simulink model "E55_1030"  (R2019b)
settings: Solver=FixedStepDiscrete  StartTime=0.0  StopTime=10  FixedStep=0.0005  RelTol=1e-3  EnableMultiTasking=on
InitFcn:
  | ecucoder_canfd
  | load('DATA_Plimit.mat')
  | a=0.775;
  | b=0.775;
  | kf=-50000;
  | kr=-50000;
  | m=226+75;
  | Iz=100;
  | u=0.85;
  | g=9.8;
  | L=a+b;
  | xi=0.1;
  | r=0.226;
  | Lw=1.171;
  | Tm=21;
  | i=15.9;
  | Jw=0.504;
  | Pmax=20000;
  | mw=19.3;
  | mb=148.9+75;
  | hg=0.280;
model workspace (MAT data in the model file):
  Initial_Steer_Position = 0
values from neighbouring files (symbols this model uses):
  SOC = [2.5 5 7.5 10 20 30 40 50 60 70 80 90 ... (14 elements, 14x1)]    [DATA_Plimit.mat]
  SOC_Discharge = [2.04592350211 2.57821618825 3.10671863859 3.63118835861 4.15200192786 4.66837694959 5.18149950051 5.69046162564 6.19532286188 6.696400261 7.19347596839 7.68712157998 ... (473 elements, 1x473)]    [DATA_Plimit.mat]
  VOLTAGE = [459.1488 476.0844 485.9448 487.344 492.822 498.8016 503.382 509.1108 518.8128 531.2472 544.5132 558.4656 ... (14 elements, 14x1)]    [DATA_Plimit.mat]
undefined symbols (not defined in the file or in its folder): DiscIntNeverNeededParam, H, HALL10, HALL6, HALL7, HALL8, HALL9, HPWM1, HPWM3, I_AN05_5V, I_AN07_5V, I_AN08_5V, I_AN09_5V, I_AN10_5V, I_SW11_H, I_SW12_H, I_SW13_H, I_SW14_H, I_SW15_H, I_SW16_H, I_SW17_H, I_SW18_H, I_SW19_H, LS1A2, O_HS1A2, O_HS1A8
libraries: ec311lib x152, simulink x92, canmsglib x30, canfdmsglib x2
(part 4 of 6)

== system E55_1030/Function-Call Subsystem2/Subsystem11 ==
  CAN_OK : Inport
  CAN ID : Inport  Port=2
  CAN Msg : Inport  Port=3
  function : TriggerPort  TriggerType=function-call  VariantControl=(inherit)
  Enabled Subsystem : Subsystem  TreatAsAtomicUnit=on
  steer_angle_data : Outport
  wires:
  CAN_OK/1 -> Enabled Subsystem/Enable  "CAN_OK"
  CAN ID/1 -> Enabled Subsystem/1(In1)
  CAN Msg/1 -> Enabled Subsystem/2(In2)
  Enabled Subsystem/1(Angle) -> steer_angle_data/1

== system E55_1030/Function-Call Subsystem2/Subsystem12 ==
  CAN_OK : Inport
  CAN ID : Inport  Port=2
  CAN Msg : Inport  Port=3
  function : TriggerPort  TriggerType=function-call  VariantControl=(inherit)
  Bus Creator : BusCreator  Inputs=4
  Enabled Subsystem : Subsystem  TreatAsAtomicUnit=on
  285_data : Outport
  wires:
  CAN_OK/1 -> Enabled Subsystem/Enable  "CAN_OK"
  CAN ID/1 -> Enabled Subsystem/1(In1)
  CAN Msg/1 -> Enabled Subsystem/2(In2)
  Bus Creator/1 -> 285_data/1
  Enabled Subsystem/1(ErrorInfo) -> Bus Creator/1  "ErrorCode"
  Enabled Subsystem/2(TempIGBT) -> Bus Creator/2  "TempIGBT"
  Enabled Subsystem/3(TempInverter) -> Bus Creator/3  "TempInverter"
  Enabled Subsystem/4(TempMotor) -> Bus Creator/4  "TempMotor"

== system E55_1030/Function-Call Subsystem2/Subsystem15 ==
  acc_x : Inport
  acc_y : Inport  Port=2
  Mux : Mux
  Saturation : Saturate  UpperLimit=1500  LowerLimit=0
  右前载荷 : Subsystem
  右后载荷 : Subsystem
  左前载荷 : Subsystem
  左后载荷 : Subsystem
  Fz : Outport
  wires:
  [acc_x] -> 左前载荷/1(acc_x)
  [acc_y] -> 左前载荷/2(acc_y)
  Mux/1 -> Saturation/1
  [acc_x] -> 右前载荷/1(acc_x)
  [acc_y] -> 右前载荷/2(acc_y)
  [acc_x] -> 左后载荷/1(acc_x)
  [acc_y] -> 左后载荷/2(acc_y)
  [acc_x] -> 右后载荷/1(acc_x)
  [acc_y] -> 右后载荷/2(acc_y)
  左前载荷/1(Fz1) -> Mux/1
  右前载荷/1(Fz2) -> Mux/2
  左后载荷/1(Fz3) -> Mux/3
  右后载荷/1(Fz4) -> Mux/4
  acc_y/1 -> [acc_x]
  acc_x/1 -> [acc_y]
  Saturation/1 -> Fz/1

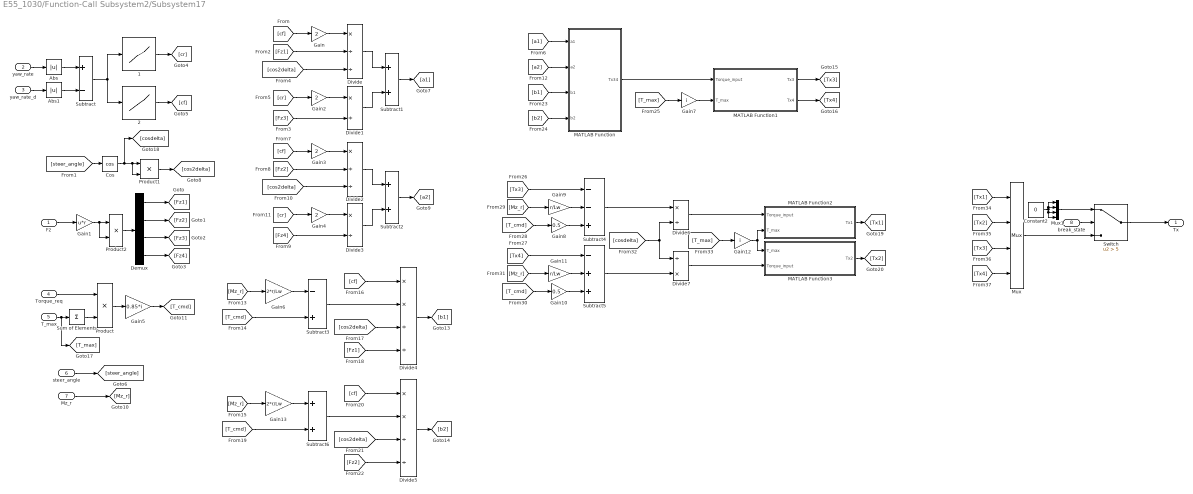
== system E55_1030/Function-Call Subsystem2/Subsystem17 ==
  Fz : Inport
  yaw_rate : Inport  Port=2
  yaw_rate_d : Inport  Port=3
  Torque_req : Inport  Port=4
  T_max : Inport  Port=5
  steer_angle : Inport  Port=6
  Mz_r : Inport  Port=7
  break_state : Inport  Port=8
  1 : Lookup_n-D  NumberOfTableDimensions=1  BreakpointsForDimension1=[-0.3,-0.2,0,0.2,0.3]  Table=[1,1,1,2,2]  InternalRulePriority=Speed  RndMeth=Simplest  InputSameDT=on
  2 : Lookup_n-D  NumberOfTableDimensions=1  BreakpointsForDimension1=[-0.3,-0.2,0,0.2,0.3]  Table=[2,2,1,1,1]  InternalRulePriority=Speed  RndMeth=Simplest  InputSameDT=on
  Abs : Abs
  Abs1 : Abs
  Constant2 : Constant  Value=0
  Cos : Trigonometry  Operator=cos
  Demux : Demux
  Divide : Product  Inputs=*//
  Divide1 : Product  Inputs=*/
  Divide2 : Product  Inputs=*//
  Divide3 : Product  Inputs=*/
  Divide4 : Product  Inputs=**//
  Divide5 : Product  Inputs=**//
  Divide6 : Product  Inputs=*/
  Divide7 : Product  Inputs=/*
  Gain{,2..4} (4 alike) : Gain  Gain=2
  Gain1 : Gain  Gain=u*r
  Gain10 : Gain  Gain=0.5
  Gain11 : Gain  Gain=r/Lw
  Gain12 : Gain  Gain=i
  Gain13 : Gain  Gain=2*r/Lw
  Gain5 : Gain  Gain=0.85*i
  Gain6 : Gain  Gain=2*r/Lw
  Gain7 : Gain  Gain=i
  Gain8 : Gain  Gain=0.5
  Gain9 : Gain  Gain=r/Lw
  MATLAB Function : MATLAB Function  TreatAsAtomicUnit=on
  MATLAB Function1 : MATLAB Function  TreatAsAtomicUnit=on
  MATLAB Function2 : MATLAB Function  TreatAsAtomicUnit=on
  MATLAB Function3 : MATLAB Function  TreatAsAtomicUnit=on
  Mux : Mux
  Mux1 : Mux
  Product : Product
  Product1 : Product
  Product2 : Product
  Subtract : Sum  Inputs=+-
  Subtract1 : Sum
  Subtract2 : Sum
  Subtract3 : Sum  Inputs=-+
  Subtract4 : Sum  Inputs=--+
  Subtract5 : Sum  Inputs=-++
  Subtract6 : Sum
  Sum of Elements : Sum  Inputs=+
  Switch : Switch  Criteria=u2 > Threshold  Threshold=5
  Tx : Outport
  wires:
  Demux/1 -> [Fz1]
  Demux/2 -> [Fz2]
  Demux/3 -> [Fz3]
  Demux/4 -> [Fz4]
  yaw_rate/1 -> Abs/1
  yaw_rate_d/1 -> Abs1/1
  Abs/1 -> Subtract/1
  Abs1/1 -> Subtract/2
  Subtract/1 -> 2/1, 1/1
  [cf] -> Gain/1
  Gain/1 -> Divide/1
  steer_angle/1 -> [steer_angle]
  [steer_angle] -> Cos/1
  [Fz1] -> Divide/2
  Cos/1 -> Product1/2, Product1/1, [cosdelta]
  Product1/1 -> [cos2delta]
  [cos2delta] -> Divide/3
  Divide/1 -> Subtract1/1
  [cr] -> Gain2/1
  Gain2/1 -> Divide1/1
  Fz/1 -> Gain1/1
  [Fz3] -> Divide1/2
  Divide1/1 -> Subtract1/2
  Subtract1/1 -> [a1]
  [a1] -> MATLAB Function/1(a1)
  Subtract2/1 -> [a2]
  Divide3/1 -> Subtract2/2
  [Fz4] -> Divide3/2
  Gain4/1 -> Divide3/1
  [cr] -> Gain4/1
  Divide2/1 -> Subtract2/1
  [cos2delta] -> Divide2/3
  [Fz2] -> Divide2/2
  Gain3/1 -> Divide2/1
  [cf] -> Gain3/1
  [a2] -> MATLAB Function/2(a2)
  Mz_r/1 -> [Mz_r]
  T_max/1 -> [T_max], Sum of Elements/1
  Torque_req/1 -> Product/1
  Product/1 -> Gain5/1
  Gain5/1 -> [T_cmd]
  [Mz_r] -> Gain6/1
  Gain6/1 -> Subtract3/1
  [T_cmd] -> Subtract3/2
  [cf] -> Divide4/1
  [cos2delta] -> Divide4/3
  [Fz1] -> Divide4/4
  Divide4/1 -> [b1]
  Divide5/1 -> [b2]
  [Fz2] -> Divide5/4
  [cos2delta] -> Divide5/3
  [cf] -> Divide5/1
  [b1] -> MATLAB Function/3(b1)
  [b2] -> MATLAB Function/4(b2)
  Sum of Elements/1 -> Product/2
  MATLAB Function/1(Tx34) -> MATLAB Function1/1(Torque_input)
  [T_max] -> Gain7/1
  Gain7/1 -> MATLAB Function1/2(T_max)
  MATLAB Function1/2(Tx4) -> [Tx4]
  MATLAB Function1/1(Tx3) -> [Tx3]
  [T_cmd] -> Gain8/1
  Gain8/1 -> Subtract4/3
  [Mz_r] -> Gain9/1
  [Tx3] -> Subtract4/1
  Gain9/1 -> Subtract4/2
  [Mz_r] -> Gain11/1
  Gain11/1 -> Subtract5/2
  Gain10/1 -> Subtract5/3
  [T_cmd] -> Gain10/1
  [Tx4] -> Subtract5/1
  Subtract4/1 -> Divide6/1
  [cosdelta] -> Divide7/1, Divide6/2
  Subtract5/1 -> Divide7/2
  Divide6/1 -> MATLAB Function2/1(Torque_input)
  [T_max] -> Gain12/1
  Gain12/1 -> MATLAB Function3/1(T_max), MATLAB Function2/2(T_max)
  Divide7/1 -> MATLAB Function3/2(Torque_input)
  MATLAB Function2/1(Tx1) -> [Tx1]
  MATLAB Function3/1(Tx2) -> [Tx2]
  Mux/1 -> Switch/3
  2/1 -> [cf]
  1/1 -> [cr]
  Subtract3/1 -> Divide4/2
  [T_cmd] -> Subtract6/2
  Gain13/1 -> Subtract6/1
  [Mz_r] -> Gain13/1
  Subtract6/1 -> Divide5/2
  break_state/1 -> Switch/2
  Switch/1 -> Tx/1
  Mux1/1 -> Switch/1
  Constant2/1 -> Mux1/3, Mux1/4, Mux1/2, Mux1/1
  [Tx1] -> Mux/1
  [Tx2] -> Mux/2
  [Tx3] -> Mux/3
  [Tx4] -> Mux/4
  Product2/1 -> Demux/1
  Gain1/1 -> Product2/2, Product2/1

== system E55_1030/Function-Call Subsystem2/Subsystem18 ==
  CAN_OK : Inport
  CAN ID : Inport  Port=2
  CAN Msg : Inport  Port=3
  DLC : Inport  Port=4
  function : TriggerPort  TriggerType=function-call  VariantControl=(inherit)
  Bus Creator : BusCreator  Inputs=7
  Enabled Subsystem : Subsystem  TreatAsAtomicUnit=on
  GNSS_data : Outport
  wires:
  CAN_OK/1 -> Enabled Subsystem/Enable, Bus Creator/1  "CAN_OK"
  CAN ID/1 -> Enabled Subsystem/1(In1)
  CAN Msg/1 -> Enabled Subsystem/2(In2)
  Bus Creator/1 -> GNSS_data/1
  DLC/1 -> Enabled Subsystem/3(In3)
  Enabled Subsystem/2(Heading_Angle) -> Bus Creator/3  "Heading_Angle"
  Enabled Subsystem/1(East_Speed) -> Bus Creator/2  "East_Speed"
  Enabled Subsystem/3(North_Speed) -> Bus Creator/4  "North_Speed"
  Enabled Subsystem/4(Pitch_Angle) -> Bus Creator/5  "Pitch_Angle"
  Enabled Subsystem/5(Roll_Angle) -> Bus Creator/6  "Roll_Angle"
  Enabled Subsystem/6(To_Ground_Speed) -> Bus Creator/7  "To_Ground_Speed"

== system E55_1030/Function-Call Subsystem2/Subsystem19 ==
  CAN_OK : Inport
  CAN ID : Inport  Port=2
  CAN Msg : Inport  Port=3
  DLC : Inport  Port=4
  function : TriggerPort  TriggerType=function-call  VariantControl=(inherit)
  Bus Creator : BusCreator  Inputs=7
  Enabled Subsystem : Subsystem  TreatAsAtomicUnit=on
  IMU_data : Outport
  wires:
  CAN_OK/1 -> Enabled Subsystem/Enable, Bus Creator/1  "CAN_OK"
  CAN ID/1 -> Enabled Subsystem/1(In1)
  CAN Msg/1 -> Enabled Subsystem/2(In2)
  Bus Creator/1 -> IMU_data/1
  DLC/1 -> Enabled Subsystem/3(In3)
  Enabled Subsystem/1(INS_IMUAccrnX) -> Bus Creator/2  "INS_IMUAccrnX"
  Enabled Subsystem/2(INS_IMUAccrnY) -> Bus Creator/3  "INS_IMUAccrnY"
  Enabled Subsystem/3(INS_IMUAccrnZ) -> Bus Creator/4  "INS_IMUAccrnZ"
  Enabled Subsystem/4(INS_IMUAglRateX) -> Bus Creator/5  "INS_IMUAglRateX"
  Enabled Subsystem/5(INS_IMUAglRateY) -> Bus Creator/6  "INS_IMUAglRateY"
  Enabled Subsystem/6(INS_IMUAglRateZ) -> Bus Creator/7  "INS_IMUAglRateZ"

== system E55_1030/Function-Call Subsystem2/Subsystem2 ==
  CAN_OK : Inport
  CAN ID : Inport  Port=2
  CAN Msg : Inport  Port=3
  function : TriggerPort  TriggerType=function-call  VariantControl=(inherit)
  Bus Creator : BusCreator  Inputs=4
  Enabled Subsystem : Subsystem  TreatAsAtomicUnit=on
  287_data : Outport
  wires:
  CAN_OK/1 -> Enabled Subsystem/Enable
  CAN ID/1 -> Enabled Subsystem/1(In1)
  CAN Msg/1 -> Enabled Subsystem/2(In2)
  Enabled Subsystem/2(287_Error) -> Bus Creator/2  "bError"
  Enabled Subsystem/1(287_ActualVelocity) -> Bus Creator/1  "AMK_Speed"
  Bus Creator/1 -> 287_data/1
  Enabled Subsystem/3(287_Id) -> Bus Creator/3  "Id"
  Enabled Subsystem/4(287_Iq) -> Bus Creator/4  "Iq"

== system E55_1030/Function-Call Subsystem2/Subsystem3 ==
  CAN_OK : Inport
  CAN ID : Inport  Port=2
  CAN Msg : Inport  Port=3
  function : TriggerPort  TriggerType=function-call  VariantControl=(inherit)
  Bus Creator : BusCreator  Inputs=4
  Enabled Subsystem : Subsystem  TreatAsAtomicUnit=on
  283_data : Outport
  wires:
  CAN_OK/1 -> Enabled Subsystem/Enable
  CAN ID/1 -> Enabled Subsystem/1(In1)
  CAN Msg/1 -> Enabled Subsystem/2(In2)
  Enabled Subsystem/2(283_Error) -> Bus Creator/2  "bError"
  Enabled Subsystem/1(283_ActualVelocity) -> Bus Creator/1  "AMK_Speed"
  Bus Creator/1 -> 283_data/1
  Enabled Subsystem/3(283_Id) -> Bus Creator/3  "Id"
  Enabled Subsystem/4(283_Iq) -> Bus Creator/4  "Iq"

== system E55_1030/Function-Call Subsystem2/Subsystem4 ==
  CAN_OK : Inport
  CAN ID : Inport  Port=2
  CAN Msg : Inport  Port=3
  function : TriggerPort  TriggerType=function-call  VariantControl=(inherit)
  Bus Creator : BusCreator  Inputs=4
  Enabled Subsystem : Subsystem  TreatAsAtomicUnit=on
  288_data : Outport
  wires:
  CAN_OK/1 -> Enabled Subsystem/Enable
  CAN ID/1 -> Enabled Subsystem/1(In1)
  CAN Msg/1 -> Enabled Subsystem/2(In2)
  Enabled Subsystem/2(288_Error) -> Bus Creator/2  "bError"
  Enabled Subsystem/1(288_ActualVelocity) -> Bus Creator/1  "AMK_Speed"
  Bus Creator/1 -> 288_data/1
  Enabled Subsystem/3(288_Id) -> Bus Creator/3  "Id"
  Enabled Subsystem/4(288_Iq) -> Bus Creator/4  "Iq"

== system E55_1030/Function-Call Subsystem2/Subsystem5 ==
  CAN_OK : Inport
  CAN ID : Inport  Port=2
  CAN Msg : Inport  Port=3
  function : TriggerPort  TriggerType=function-call  VariantControl=(inherit)
  Bus Creator : BusCreator  Inputs=4
  Enabled Subsystem : Subsystem  TreatAsAtomicUnit=on
  286_data : Outport
  wires:
  CAN_OK/1 -> Enabled Subsystem/Enable  "CAN_OK"
  CAN ID/1 -> Enabled Subsystem/1(In1)
  CAN Msg/1 -> Enabled Subsystem/2(In2)
  Bus Creator/1 -> 286_data/1
  Enabled Subsystem/1(ErrorInfo) -> Bus Creator/1  "ErrorCode"
  Enabled Subsystem/2(TempIGBT) -> Bus Creator/2  "TempIGBT"
  Enabled Subsystem/3(TempInverter) -> Bus Creator/3  "TempInverter"
  Enabled Subsystem/4(TempMotor) -> Bus Creator/4  "TempMotor"

== system E55_1030/Function-Call Subsystem2/Subsystem6 ==
  CAN_OK : Inport
  CAN ID : Inport  Port=2
  CAN Msg : Inport  Port=3
  function : TriggerPort  TriggerType=function-call  VariantControl=(inherit)
  Bus Creator : BusCreator  Inputs=4
  Enabled Subsystem : Subsystem  TreatAsAtomicUnit=on
  289_data : Outport
  wires:
  CAN_OK/1 -> Enabled Subsystem/Enable  "CAN_OK"
  CAN ID/1 -> Enabled Subsystem/1(In1)
  CAN Msg/1 -> Enabled Subsystem/2(In2)
  Bus Creator/1 -> 289_data/1
  Enabled Subsystem/1(ErrorInfo) -> Bus Creator/1  "ErrorCode"
  Enabled Subsystem/2(TempIGBT) -> Bus Creator/2  "TempIGBT"
  Enabled Subsystem/3(TempInverter) -> Bus Creator/3  "TempInverter"
  Enabled Subsystem/4(TempMotor) -> Bus Creator/4  "TempMotor"

== system E55_1030/Function-Call Subsystem2/Subsystem7 ==
  CAN_OK : Inport
  CAN ID : Inport  Port=2
  CAN Msg : Inport  Port=3
  function : TriggerPort  TriggerType=function-call  VariantControl=(inherit)
  Bus Creator : BusCreator  Inputs=4
  Enabled Subsystem : Subsystem  TreatAsAtomicUnit=on
  28A_data : Outport
  wires:
  CAN_OK/1 -> Enabled Subsystem/Enable  "CAN_OK"
  CAN ID/1 -> Enabled Subsystem/1(In1)
  CAN Msg/1 -> Enabled Subsystem/2(In2)
  Bus Creator/1 -> 28A_data/1
  Enabled Subsystem/1(ErrorInfo) -> Bus Creator/1  "ErrorCode"
  Enabled Subsystem/2(TempIGBT) -> Bus Creator/2  "TempIGBT"
  Enabled Subsystem/3(TempInverter) -> Bus Creator/3  "TempInverter"
  Enabled Subsystem/4(TempMotor) -> Bus Creator/4  "TempMotor"

== system E55_1030/Function-Call Subsystem2/Subsystem8 ==
  CAN_OK : Inport
  CAN ID : Inport  Port=2
  CAN Msg : Inport  Port=3
  function : TriggerPort  TriggerType=function-call  VariantControl=(inherit)
  Bus Creator : BusCreator  Inputs=2
  Enabled Subsystem : Subsystem  TreatAsAtomicUnit=on
  IVT_data : Outport
  wires:
  CAN_OK/1 -> Enabled Subsystem/Enable  "CAN_OK"
  CAN ID/1 -> Enabled Subsystem/1(In1)
  CAN Msg/1 -> Enabled Subsystem/2(In2)
  Bus Creator/1 -> IVT_data/1
  Enabled Subsystem/1(IVT_MsgCount) -> Bus Creator/1  "IVT_MsgCount"
  Enabled Subsystem/2(IVT_Msg_Result_W) -> Bus Creator/2  "IVT_Msg_Result_W"

== system E55_1030/Function-Call Subsystem2/Triggered Subsystem ==
  Trigger : TriggerPort  TriggerType=falling  VariantControl=Variant
  AMK_Setpoints_Motor1 : Subsystem
  AMK_Setpoints_Motor2 : Subsystem
  AMK_Setpoints_Motor3 : Subsystem
  AMK_Setpoints_Motor4 : Subsystem
  Constant{,1..3} (4 alike) : Constant  Value=0
  Constant{4..6,15} (4 alike) : Constant  Value=1792
  Terminator{42..43,48,50} (4 alike) : Terminator
  右前 : ec311lib/RapidECU_U34/03CANCommunication/CAN0to2Transmit  canmodule=2  canbuffer=8  canmessageid=hex2dec('0185')  canmessagetype=Standard(11-bit ID)  datalength=8  sampletime=-1
      settings: SourceProductName=ECUCoder for S32K311
  右后 : ec311lib/RapidECU_U34/03CANCommunication/CAN0to2Transmit  canmodule=2  canbuffer=11  canmessageid=hex2dec('0189')  canmessagetype=Standard(11-bit ID)  datalength=8  sampletime=-1
      settings: SourceProductName=ECUCoder for S32K311
  左前 : ec311lib/RapidECU_U34/03CANCommunication/CAN0to2Transmit  canmodule=2  canbuffer=7  canmessageid=hex2dec('0184')  canmessagetype=Standard(11-bit ID)  datalength=8  sampletime=-1
      settings: SourceProductName=ECUCoder for S32K311
  左后 : ec311lib/RapidECU_U34/03CANCommunication/CAN0to2Transmit  canmodule=2  canbuffer=10  canmessageid=hex2dec('0188')  canmessagetype=Standard(11-bit ID)  datalength=8  sampletime=-1
      settings: SourceProductName=ECUCoder for S32K311
  wires:
  AMK_Setpoints_Motor1/1(output) -> 右前/1
  AMK_Setpoints_Motor3/1(output) -> 左前/1
  右前/1 -> Terminator42/1
  左后/1 -> Terminator48/1
  AMK_Setpoints_Motor2/1(output) -> 左后/1
  左前/1 -> Terminator43/1
  AMK_Setpoints_Motor4/1(output) -> 右后/1
  右后/1 -> Terminator50/1
  Constant/1 -> AMK_Setpoints_Motor1/3(AMK_TargetVelocity_in), AMK_Setpoints_Motor1/1(AMK_TorqueLimitNegativ_in), AMK_Setpoints_Motor1/2(AMK_TorqueLimitPositiv_in)
  Constant1/1 -> AMK_Setpoints_Motor3/3(AMK_TargetVelocity_in), AMK_Setpoints_Motor3/2(AMK_TorqueLimitPositiv_in), AMK_Setpoints_Motor3/1(AMK_TorqueLimitNegativ_in)
  Constant2/1 -> AMK_Setpoints_Motor4/2(AMK_TorqueLimitPositiv_in), AMK_Setpoints_Motor4/3(AMK_TargetVelocity_in), AMK_Setpoints_Motor4/1(AMK_TorqueLimitNegativ_in)
  Constant3/1 -> AMK_Setpoints_Motor2/3(AMK_TargetVelocity_in), AMK_Setpoints_Motor2/2(AMK_TorqueLimitPositiv_in), AMK_Setpoints_Motor2/1(AMK_TorqueLimitNegativ_in)
  Constant15/1 -> AMK_Setpoints_Motor1/4(AMK_Control_in)
  Constant4/1 -> AMK_Setpoints_Motor2/4(AMK_Control_in)
  Constant5/1 -> AMK_Setpoints_Motor3/4(AMK_Control_in)
  Constant6/1 -> AMK_Setpoints_Motor4/4(AMK_Control_in)

== system E55_1030/Function-Call Subsystem2/功率限制 ==
  MaxTempMotor : Inport
  wheel_speed : Inport  Port=2
  "Power " : Inport  Port=3
  1-D Lookup Table1 : Lookup_n-D  NumberOfTableDimensions=1  BreakpointsForDimension1=[0;80;100;120]  Table=[22.3056525;22.3056525;21.8349456;21.3643326]  InternalRulePriority=Speed  RndMeth=Simplest  InputSameDT=on
  Constant : Constant  Value=60/(2*pi)
  Divide1 : Product  Inputs=**/
  Min : MinMax  Inputs=2
  Saturation : Saturate  UpperLimit=20000  LowerLimit=2000
  T_max : Outport
  wires:
  MaxTempMotor/1 -> 1-D Lookup Table1/1
  Divide1/1 -> Min/1
  Min/1 -> T_max/1
  wheel_speed/1 -> Saturation/1
  [T_max_temp] -> Min/2
  1-D Lookup Table1/1 -> [T_max_temp]
  Constant/1 -> Divide1/2
  "Power "/1 -> Divide1/1
  Saturation/1 -> Divide1/3

== system E55_1030/Function-Call Subsystem2/功率限制1 ==
  MaxTempMotor : Inport
  wheel_speed : Inport  Port=2
  DeratingRatio : Inport  Port=3
  1-D Lookup Table1 : Lookup_n-D  NumberOfTableDimensions=1  BreakpointsForDimension1=[0;80;100;120]  Table=[22.3056525;22.3056525;21.8349456;21.3643326]  InternalRulePriority=Speed  RndMeth=Simplest  InputSameDT=on
  Constant : Constant  Value=60*20000/(2*pi)
  Divide1 : Product  Inputs=*/
  Gain : Gain  Gain=i
  Min : MinMax  Inputs=2
  Product : Product
  Saturation : Saturate  UpperLimit=20000  LowerLimit=5000
  T_max : Outport
  wires:
  MaxTempMotor/1 -> 1-D Lookup Table1/1
  Divide1/1 -> Min/1
  Gain/1 -> Saturation/1
  [T_max_temp] -> Min/2
  1-D Lookup Table1/1 -> [T_max_temp]
  Constant/1 -> Divide1/1
  wheel_speed/1 -> Gain/1
  Min/1 -> Product/1
  DeratingRatio/1 -> Product/2
  Product/1 -> T_max/1
  Saturation/1 -> Divide1/2

== system E55_1030/Function-Call Subsystem2/计算最大驱动力 ==
  torque : Inport
  wheel_speed : Inport  Port=2
  Add : Sum  Inputs=+-
  Discrete Derivative : simulink/Discrete/Discrete Derivative  gainval=1.0  ICPrevScaledInput=0.0  OutMin=[]  OutMax=[]  OutDataType=fixdt(1, 16)  OutScaling=2^-10  DoSatur=off
  Gain : Gain  Gain=Jw
  Gain1 : Gain  Gain=2*pi/60
  Gain4 : Gain  Gain=1/r
  Saturation : Saturate  UpperLimit=330  LowerLimit=-330
  Fx_max : Outport
  wires:
  Saturation/1 -> Add/2
  Gain4/1 -> Fx_max/1
  Discrete Derivative/1 -> Gain/1
  Gain/1 -> Saturation/1
  torque/1 -> Add/1
  Add/1 -> Gain4/1
  wheel_speed/1 -> Gain1/1
  Gain1/1 -> Discrete Derivative/1

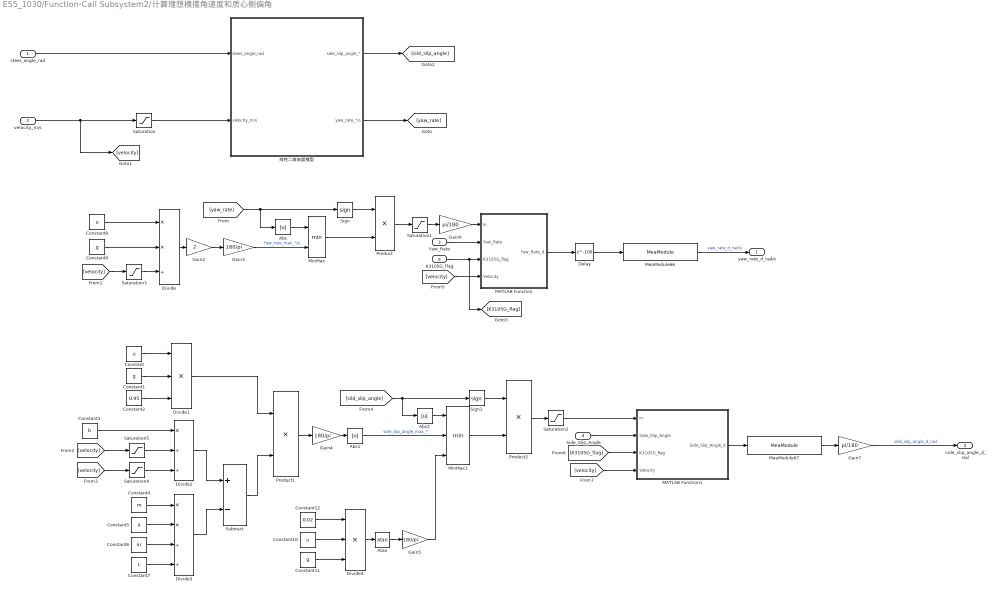
== system E55_1030/Function-Call Subsystem2/计算理想横摆角速度和质心侧偏角 ==
  steer_angle_rad : Inport
  velocity_m/s : Inport  Port=2
  Yaw_Rate : Inport  Port=3
  Side_Slip_Angle : Inport  Port=4
  K3105G_flag : Inport  Port=5
  Abs : Abs
  Abs1 : Abs
  Abs2 : Abs
  Atan : Trigonometry  Operator=atan
  Constant : Constant  Value=u
  Constant1 : Constant  Value=g
  Constant10 : Constant  Value=u
  Constant11 : Constant  Value=g
  Constant12 : Constant  Value=0.02
  Constant2 : Constant  Value=0.95
  Constant3 : Constant  Value=b
  Constant4 : Constant  Value=m
  Constant5 : Constant  Value=a
  Constant6 : Constant  Value=kr
  Constant7 : Constant  Value=L
  Constant8 : Constant  Value=u
  Constant9 : Constant  Value=g
  Delay : Delay  DelayLength=100
  Divide : Product  Inputs=**/
  Divide1 : Product  Inputs=***
  Divide2 : Product  Inputs=*//
  Divide3 : Product  Inputs=**//
  Divide4 : Product  Inputs=***
  Gain2 : Gain  Gain=2
  Gain3 : Gain  Gain=180/pi
  Gain4 : Gain  Gain=180/pi
  Gain5 : Gain  Gain=180/pi
  Gain6 : Gain  Gain=pi/180
  Gain7 : Gain  Gain=pi/180
  MATLAB Function : MATLAB Function  TreatAsAtomicUnit=on
  MATLAB Function1 : MATLAB Function  TreatAsAtomicUnit=on
  MeaModule66 : ec311lib/RapidECU_U34/09Calibration/MeaModule  signal=Yaw_Rate_d
      settings: SourceProductName=ECUCoder for S32K311
  MeaModule67 : ec311lib/RapidECU_U34/09Calibration/MeaModule  signal=Side_Slip_Angle_d
      settings: SourceProductName=ECUCoder for S32K311
  MinMax : MinMax  Inputs=2
  MinMax1 : MinMax  Inputs=3
  Product : Product
  Product1 : Product
  Product2 : Product
  Saturation{,3..5} (4 alike) : Saturate  UpperLimit=120  LowerLimit=5/3.6
  Saturation1 : Saturate  UpperLimit=120  LowerLimit=-120
  Saturation2 : Saturate  UpperLimit=30  LowerLimit=-30
  Sign : Signum
  Sign1 : Signum
  Subtract : Sum  Inputs=+-
  线性二自由度模型 : Subsystem
  yaw_rate_d_rad/s : Outport
  side_slip_angle_d_rad : Outport  Port=2
  wires:
  [yaw_rate] -> Abs/1, Sign/1
  Constant8/1 -> Divide/1
  Divide2/1 -> Subtract/1
  Constant4/1 -> Divide3/1
  steer_angle_rad/1 -> 线性二自由度模型/1(steer_angle_rad)
  Constant2/1 -> Divide1/3
  Product2/1 -> Saturation2/1
  线性二自由度模型/2(yaw_rate_°/s) -> [yaw_rate]
  [sild_slip_angle] -> Sign1/1, Abs2/1
  [velocity] -> Saturation3/1
  Constant/1 -> Divide1/1
  Constant3/1 -> Divide2/1
  Sign1/1 -> Product2/1
  [velocity] -> Saturation5/1
  Sign/1 -> Product/1
  Gain2/1 -> Gain3/1
  Constant1/1 -> Divide1/2
  Divide1/1 -> Product1/1
  velocity_m/s/1 -> [velocity], Saturation/1
  [velocity] -> Saturation4/1
  Divide3/1 -> Subtract/2
  Constant6/1 -> Divide3/3
  Subtract/1 -> Product1/2
  Constant5/1 -> Divide3/2
  MinMax1/1 -> Product2/2
  Product1/1 -> Gain4/1
  Divide/1 -> Gain2/1
  Constant7/1 -> Divide3/4
  Abs2/1 -> MinMax1/1
  Saturation/1 -> 线性二自由度模型/2(velocity_m/s)
  Constant9/1 -> Divide/2
  Gain4/1 -> Abs1/1
  线性二自由度模型/1(side_slip_angle_°) -> [sild_slip_angle]
  Product/1 -> Saturation1/1
  Constant10/1 -> Divide4/2
  Constant11/1 -> Divide4/3
  Constant12/1 -> Divide4/1
  Divide4/1 -> Atan/1
  Atan/1 -> Gain5/1
  Gain5/1 -> MinMax1/3
  Gain7/1 -> side_slip_angle_d_rad/1  "side_slip_angle_d_rad"
  Abs1/1 -> MinMax1/2  "side_slip_angle_max_°"
  Abs/1 -> MinMax/1
  MinMax/1 -> Product/2
  Gain3/1 -> MinMax/2  "Yaw_rate_max_°/s"
  MeaModule67/1 -> Gain7/1
  Saturation1/1 -> Gain6/1
  Yaw_Rate/1 -> MATLAB Function/2(Yaw_Rate)
  K3105G_flag/1 -> [K3105G_flag], MATLAB Function/3(K3105G_flag)
  MATLAB Function/1(Yaw_Rate_d) -> Delay/1
  [velocity] -> MATLAB Function/4(Velocity)
  Saturation2/1 -> MATLAB Function1/1(in)
  Side_Slip_Angle/1 -> MATLAB Function1/2(Side_Slip_Angle)
  [K3105G_flag] -> MATLAB Function1/3(K3105G_flag)
  [velocity] -> MATLAB Function1/4(Velocity)
  MATLAB Function1/1(Side_Slip_Angle_d) -> MeaModule67/1
  Gain6/1 -> MATLAB Function/1(in)
  MeaModule66/1 -> yaw_rate_d_rad/s/1  "yaw_rate_d_rad/s"
  Saturation3/1 -> Divide/3
  Saturation4/1 -> Divide2/3
  Saturation5/1 -> Divide2/2
  Delay/1 -> MeaModule66/1

== system E55_1030/Function-Call Subsystem2/计算理想转速 ==
  velocity : Inport
  Yaw_Rate : Inport  Port=2
  steer_angle : Inport  Port=3
  Gain{,1..3} (4 alike) : Gain  Gain=60/(2*pi)
  MeaModule : ec311lib/RapidECU_U34/09Calibration/MeaModule  signal=wheel_speed_d_fr
      settings: SourceProductName=ECUCoder for S32K311
  MeaModule1 : ec311lib/RapidECU_U34/09Calibration/MeaModule  signal=wheel_speed_d_fl
      settings: SourceProductName=ECUCoder for S32K311
  MeaModule2 : ec311lib/RapidECU_U34/09Calibration/MeaModule  signal=wheel_speed_d_rr
      settings: SourceProductName=ECUCoder for S32K311
  MeaModule3 : ec311lib/RapidECU_U34/09Calibration/MeaModule  signal=wheel_speed_d_rl
      settings: SourceProductName=ECUCoder for S32K311
  Mux2 : Mux
  Saturation{,1..3} (4 alike) : Saturate  UpperLimit=1500  LowerLimit=0
  计算右前理想转速 : Subsystem
  计算右后理想转速 : Subsystem
  计算左前理想转速 : Subsystem
  计算左后理想转速 : Subsystem
  wheel_speed_d : Outport
  wires:
  Yaw_Rate/1 -> 计算左后理想转速/2(Yaw_Rate), 计算右后理想转速/2(Yaw_Rate), 计算右前理想转速/2(Yaw_Rate), 计算左前理想转速/2(Yaw_Rate)
  计算右后理想转速/1(wheel_speed_d_rr) -> Saturation2/1
  计算左前理想转速/1(wheel_speed_d_fl) -> Saturation1/1
  计算左后理想转速/1(wheel_speed_d_rl) -> Saturation3/1
  steer_angle/1 -> 计算右前理想转速/3(steer_angle), 计算左前理想转速/3(steer_angle)
  velocity/1 -> 计算右前理想转速/1(velocity), 计算左后理想转速/1(velocity), 计算右后理想转速/1(velocity), 计算左前理想转速/1(velocity)
  计算右前理想转速/1(wheel_speed_d_fr) -> Saturation/1
  Mux2/1 -> wheel_speed_d/1
  MeaModule/1 -> Mux2/1
  MeaModule1/1 -> Mux2/2
  MeaModule2/1 -> Mux2/3
  MeaModule3/1 -> Mux2/4
  Gain/1 -> MeaModule/1
  Gain1/1 -> MeaModule1/1
  Gain2/1 -> MeaModule2/1
  Gain3/1 -> MeaModule3/1
  Saturation/1 -> Gain/1
  Saturation1/1 -> Gain1/1
  Saturation2/1 -> Gain2/1
  Saturation3/1 -> Gain3/1

== system E55_1030/Function-Call Subsystem2/驱动防滑使能 ==
  Torque_ASR : Inport
  wheel_speed : Inport  Port=2
  wheel_speed_d : Inport  Port=3
  Torque : Inport  Port=4
  MATLAB Function : MATLAB Function  TreatAsAtomicUnit=on
  Saturation : Saturate  UpperLimit=1500  LowerLimit=5
  Switch : Switch  Criteria=u2 > Threshold  Threshold=0.1
  Torque_Out : Outport
  ASR_Status : Outport  Port=2
  wires:
  Torque_ASR/1 -> Switch/1
  MATLAB Function/1(s) -> ASR_Status/1, Switch/2
  Torque/1 -> Switch/3
  wheel_speed/1 -> Saturation/1
  wheel_speed_d/1 -> MATLAB Function/2(wheel_speed_d)
  Saturation/1 -> MATLAB Function/1(wheel_speed)
  Switch/1 -> Torque_Out/1

== system E55_1030/Function-Call Subsystem3/If Action Subsystem ==
  CAN0 0x111 BMS CAN发送 : Inport
  Action Port : ActionPort  ActionPortLabel=if(u1 >= 10)
  BMS状态控制（控制BMS是否处于Driving状态） : ec311lib/RapidECU_U34/03CANCommunication/CAN0to2Transmit  canmodule=0  canbuffer=15  canmessageid=hex2dec('0111')  canmessagetype=Standard(11-bit ID)  datalength=1  sampletime=-1
      settings: SourceProductName=ECUCoder for S32K311
  Terminator1 : Terminator
  wires:
  CAN0 0x111 BMS CAN发送/1 -> BMS状态控制（控制BMS是否处于Driving状态）/1
  BMS状态控制（控制BMS是否处于Driving状态）/1 -> Terminator1/1

== system E55_1030/Function-Call Subsystem2/Function-Call Subsystem/Enabled Subsystem ==
  CAN_ID : Inport
  CAN_MSG : Inport  Port=2
  Enable : EnablePort
  CAN Unpack : canmsglib/CAN Unpack  MsgList=(none)  MsgName=Dashboard_Control  MsgIDType=Standard (11-bit identifier)  MsgIdentifier=1374  MsgLength=8  SignalInfo={ 'K3105_Alive', '0', '1', 'LE', 'signed', 'Standard', '0', '1', '0', '0', '1' }  IDPort=off  TimestampPort=off  ErrorPort=off  RemotePort=off  LengthPort=off  StatusPort=off  ApplyMinMax=off
      settings: SourceProductName=Vehicle Network Toolbox  SourceProductBaseCode=VN
  CANUnPackMessage : ec311lib/RapidECU_U34/03CANCommunication/CANUnPackMessage  datalength=8  canmessagetype=Standard(11-bit ID)  sampletime=-1
      settings: SourceProductName=ECUCoder for S32K311
  K3105_Alive : Outport
  wires:
  CAN_ID/1 -> CANUnPackMessage/1
  CAN_MSG/1 -> CANUnPackMessage/2
  CANUnPackMessage/1 -> CAN Unpack/1
  CAN Unpack/1 -> K3105_Alive/1

== system E55_1030/Function-Call Subsystem2/SMC_yaw_rate/sat ==
  s : Inport
  Abs : Abs
  Gain1 : Gain  Gain=1/0.5
  Sign : Signum
  Switch : Switch  Criteria=u2 > Threshold  Threshold=0.5
  sat(s) : Outport
  wires:
  Switch/1 -> sat(s)/1
  Sign/1 -> Switch/1
  Gain1/1 -> Switch/3
  Abs/1 -> Switch/2
  s/1 -> Gain1/1, Abs/1, Sign/1

== system E55_1030/Function-Call Subsystem2/SMC_yaw_rate/sat1 ==
  s : Inport
  Abs : Abs
  Gain1 : Gain  Gain=1/0.035
  Sign : Signum
  Switch : Switch  Criteria=u2 > Threshold  Threshold=0.035
  sat(s) : Outport
  wires:
  s/1 -> Abs/1
  Gain1/1 -> Switch/3
  Sign/1 -> Switch/1
  Switch/1 -> sat(s)/1
  Abs/1 -> Switch/2, Sign/1, Gain1/1

== system E55_1030/Function-Call Subsystem2/Subsystem1/Enabled Subsystem ==
  In1 : Inport
  In2 : Inport  Port=2
  Enable : EnablePort
  CAN Unpack : canmsglib/CAN Unpack  MsgList=(none)  MsgName=MCU4_284  MsgIDType=Standard (11-bit identifier)  MsgIdentifier=644  MsgLength=8  SignalInfo={ 'MCU4_288_ActualVelocity', '16', '16', 'LE', 'signed', 'Standard', '0', '1', '0', '-32768', '32767'; 'MCU4_288_Error', '9', '1', 'LE', 'unsigned', 'Standard', '0', '1', '0', '0', '1'; 'MCU4_288_ManetizingCurrent', '48', '16', 'LE', 'signed', 'Standard', '0', '0.001', '0', '-20', '20'; 'MCU4_288_TorqueCurrent', '32', '16', 'LE', 'signed', 'Standard', '0', '0.001', '0', '-20', '20' }  IDPort=off  TimestampPort=off  ErrorPort=off  RemotePort=off  LengthPort=off  StatusPort=off  ApplyMinMax=off
      settings: SourceProductName=Vehicle Network Toolbox  SourceProductBaseCode=VN
  CANUnPackMessage : ec311lib/RapidECU_U34/03CANCommunication/CANUnPackMessage  datalength=8  canmessagetype=Standard(11-bit ID)  sampletime=-1
      settings: SourceProductName=ECUCoder for S32K311
  284_ActualVelocity : Outport
  284_Error : Outport  Port=2
  284_Id : Outport  Port=3
  284_Iq : Outport  Port=4
  wires:
  CANUnPackMessage/1 -> CAN Unpack/1
  In2/1 -> CANUnPackMessage/2
  In1/1 -> CANUnPackMessage/1
  CAN Unpack/1 -> 284_ActualVelocity/1
  CAN Unpack/2 -> 284_Error/1
  CAN Unpack/3 -> 284_Id/1
  CAN Unpack/4 -> 284_Iq/1

== system E55_1030/Function-Call Subsystem2/Subsystem10/Enabled Subsystem ==
  In1 : Inport
  In2 : Inport  Port=2
  Enable : EnablePort
  CAN Unpack10 : canmsglib/CAN Unpack  MsgList=(none)  MsgName=BMS_To_Driver  MsgIDType=Standard (11-bit identifier)  MsgIdentifier=1370  MsgLength=8  SignalInfo={ 'BMS_State', '16', '8', 'LE', 'unsigned', 'Standard', '0', '1', '0', '0', '255'; 'MaxCellTemp', '0', '16', 'LE', 'unsigned', 'Standard', '0', '0.1', '0', '-Inf', 'Inf'; 'MaxCellVolt', '40', '8', 'LE', 'unsigned', 'Standard', '0', '0.1', '0', '-Inf', 'Inf'; 'MinCellVolt', '24', '13', 'LE', 'unsigned', 'Standard', '0', '0.001', '0', '0', '4.35'; 'SOC', '48', '16', 'LE', 'unsigned', 'Standard', '0', '0.01', '0', '-Inf', 'Inf' }  IDPort=off  TimestampPort=off  ErrorPort=off  RemotePort=off  LengthPort=off  StatusPort=off  ApplyMinMax=off
      settings: SourceProductName=Vehicle Network Toolbox  SourceProductBaseCode=VN
  CANUnPackMessage10 : ec311lib/RapidECU_U34/03CANCommunication/CANUnPackMessage  datalength=8  canmessagetype=Standard(11-bit ID)  sampletime=-1
      settings: SourceProductName=ECUCoder for S32K311
  BMSState : Outport
  CellTemp : Outport  Port=2
  MaxCellVolt : Outport  Port=3
  MinCellVolt : Outport  Port=4
  SOC : Outport  Port=5
  wires:
  In2/1 -> CANUnPackMessage10/2
  In1/1 -> CANUnPackMessage10/1
  CANUnPackMessage10/1 -> CAN Unpack10/1
  CAN Unpack10/1 -> BMSState/1
  CAN Unpack10/2 -> CellTemp/1
  CAN Unpack10/3 -> MaxCellVolt/1
  CAN Unpack10/4 -> MinCellVolt/1
  CAN Unpack10/5 -> SOC/1

== system E55_1030/Function-Call Subsystem2/Subsystem11/Enabled Subsystem ==
  In1 : Inport
  In2 : Inport  Port=2
  Enable : EnablePort
  CAN Unpack8 : canmsglib/CAN Unpack  CANdbFile=J:\A_Home\Code\DBC\方向盘转角传感器.dbc  MsgList=Angle  MsgName=Angle  MsgIDType=Standard (11-bit identifier)  MsgIdentifier=485  MsgLength=8  SignalInfo={'Angle','16','16','BE','signed','Standard','0','0.0625','0','-900','900'}  IDPort=off  TimestampPort=off  ErrorPort=off  RemotePort=off  LengthPort=off  StatusPort=off  ApplyMinMax=off
      settings: SourceProductName=Vehicle Network Toolbox  SourceProductBaseCode=VN  DataFormat=CANdb specified signals
  CANUnPackMessage9 : ec311lib/RapidECU_U34/03CANCommunication/CANUnPackMessage  datalength=8  canmessagetype=Standard(11-bit ID)  sampletime=-1
      settings: SourceProductName=ECUCoder for S32K311
  Angle : Outport
  wires:
  In2/1 -> CANUnPackMessage9/2
  In1/1 -> CANUnPackMessage9/1
  CANUnPackMessage9/1 -> CAN Unpack8/1
  CAN Unpack8/1 -> Angle/1

== system E55_1030/Function-Call Subsystem2/Subsystem12/Enabled Subsystem ==
  In1 : Inport
  In2 : Inport  Port=2
  Enable : EnablePort
  CAN Unpack4 : canmsglib/CAN Unpack  MsgList=(none)  MsgName=MCU4_285  MsgIDType=Standard (11-bit identifier)  MsgIdentifier=645  MsgLength=8  SignalInfo={ 'MCU4_285_ErrorInfo', '32', '16', 'LE', 'unsigned', 'Standard', '0', '1', '0', '0', '65535'; 'MCU4_285_TempIGBT', '48', '16', 'LE', 'signed', 'Standard', '0', '0.1', '0', '-3276.8', '3276.7'; 'MCU4_285_TempInverter', '16', '16', 'LE', 'signed', 'Standard', '0', '0.1', '0', '-3276.8', '3276.7'; 'MCU4_285_TempMotor', '0', '16', 'LE', 'signed', 'Standard', '0', '0.1', '0', '-3276.8', '3276.7' }  IDPort=off  TimestampPort=off  ErrorPort=off  RemotePort=off  LengthPort=off  StatusPort=off  ApplyMinMax=off
      settings: SourceProductName=Vehicle Network Toolbox  SourceProductBaseCode=VN
  CANUnPackMessage4 : ec311lib/RapidECU_U34/03CANCommunication/CANUnPackMessage  datalength=8  canmessagetype=Standard(11-bit ID)  sampletime=-1
      settings: SourceProductName=ECUCoder for S32K311
  ErrorInfo : Outport
  TempIGBT : Outport  Port=2
  TempInverter : Outport  Port=3
  TempMotor : Outport  Port=4
  wires:
  In2/1 -> CANUnPackMessage4/2
  In1/1 -> CANUnPackMessage4/1
  CAN Unpack4/1 -> ErrorInfo/1
  CAN Unpack4/2 -> TempIGBT/1
  CANUnPackMessage4/1 -> CAN Unpack4/1
  CAN Unpack4/4 -> TempMotor/1
  CAN Unpack4/3 -> TempInverter/1

== system E55_1030/Function-Call Subsystem2/Subsystem15/右前载荷 ==
  acc_x : Inport
  acc_y : Inport  Port=2
  Constant : Constant  Value=mw*g+0.5*mb*g*b/L
  Gain : Gain  Gain=0.5*mb*hg/L
  Gain1 : Gain  Gain=0.5*mb*hg/Lw
  Subtract : Sum  Inputs=+++
  Fz2 : Outport
  wires:
  acc_x/1 -> Gain/1
  Gain/1 -> Subtract/2
  Constant/1 -> Subtract/1
  acc_y/1 -> Gain1/1
  Gain1/1 -> Subtract/3
  Subtract/1 -> Fz2/1

== system E55_1030/Function-Call Subsystem2/Subsystem15/右后载荷 ==
  acc_x : Inport
  acc_y : Inport  Port=2
  Constant : Constant  Value=mw*g+0.5*mb*g*a/L
  Gain : Gain  Gain=0.5*mb*hg/L
  Gain1 : Gain  Gain=0.5*mb*hg/Lw
  Subtract : Sum  Inputs=+-+
  Fz4 : Outport
  wires:
  acc_x/1 -> Gain/1
  Gain/1 -> Subtract/2
  Constant/1 -> Subtract/1
  acc_y/1 -> Gain1/1
  Gain1/1 -> Subtract/3
  Subtract/1 -> Fz4/1

== system E55_1030/Function-Call Subsystem2/Subsystem15/左前载荷 ==
  acc_x : Inport
  acc_y : Inport  Port=2
  Constant : Constant  Value=mw*g+0.5*mb*g*b/L
  Gain : Gain  Gain=0.5*mb*hg/L
  Gain1 : Gain  Gain=0.5*mb*hg/Lw
  Subtract : Sum  Inputs=++-
  Fz1 : Outport
  wires:
  acc_x/1 -> Gain/1
  Gain/1 -> Subtract/2
  Constant/1 -> Subtract/1
  acc_y/1 -> Gain1/1
  Gain1/1 -> Subtract/3
  Subtract/1 -> Fz1/1

== system E55_1030/Function-Call Subsystem2/Subsystem15/左后载荷 ==
  acc_x : Inport
  acc_y : Inport  Port=2
  Constant : Constant  Value=mw*g+0.5*mb*g*a/L
  Gain : Gain  Gain=0.5*mb*hg/L
  Gain1 : Gain  Gain=0.5*mb*hg/Lw
  Subtract : Sum  Inputs=+--
  Fz3 : Outport
  wires:
  acc_x/1 -> Gain/1
  Gain/1 -> Subtract/2
  Constant/1 -> Subtract/1
  acc_y/1 -> Gain1/1
  Gain1/1 -> Subtract/3
  Subtract/1 -> Fz3/1

== system E55_1030/Function-Call Subsystem2/Subsystem18/Enabled Subsystem ==
  In1 : Inport
  In2 : Inport  Port=2
  In3 : Inport  Port=3
  Enable : EnablePort
  CAN FD Unpack : canfdmsglib/CAN FD Unpack  MsgList=(none)  MsgName=INS_3_GNSS  ProtocolMode=CAN FD  MsgIDType=Standard (11-bit identifier)  MsgIdentifier=253  MsgLength=64  SignalInfo={ 'INS_EastSpd', '152', '16', 'BE', 'unsigned', 'Standard', '0', '0.0030517', '-100', '-100', '99.9901'; 'INS_Headg', '296', '16', 'BE', 'unsigned', 'Standard', '0', '0.010987', '-360', '0', '360'; 'INS_NorthSpd', '168', '16', 'BE', 'unsigned', 'Standard', '0', '0.0030517', '-100', '-100', '99.9901'; 'INS_Pitch', '360', '16', 'BE', 'unsigned', 'Standard', '0', '0.010987', '-360', '-180', '180'; 'INS_Roll', '416', '16', 'BE', 'unsigned', 'Standard', '0', '0.010987', '-360', '-180', '180'; 'INS_ToGndSpd', '136', '16', 'BE', 'unsigned', 'Standard', '0', '0.0030517', '-100', '-100', '99.9901' }  IDPort=off  TimestampPort=off  ErrorPort=off  RemotePort=off  LengthPort=off  StatusPort=off  BRSPort=off  ESIPort=off  DLCPort=off  ApplyMinMax=off
      settings: SourceProductName=Vehicle Network Toolbox  SourceProductBaseCode=VN  DataFormat=manually specified signals
  CANFDUnPackMessage : ec311lib/RapidECU_U34/04CANFDCommunication/CANFDUnPackMessage  mtype=0
      settings: SourceProductName=ECUCoder for S32K311
  East_Speed : Outport
  Heading_Angle : Outport  Port=2
  North_Speed : Outport  Port=3
  Pitch_Angle : Outport  Port=4
  Roll_Angle : Outport  Port=5
  To_Ground_Speed : Outport  Port=6
  wires:
  In1/1 -> CANFDUnPackMessage/1
  In2/1 -> CANFDUnPackMessage/2
  In3/1 -> CANFDUnPackMessage/3
  CANFDUnPackMessage/1 -> CAN FD Unpack/1
  CAN FD Unpack/2 -> Heading_Angle/1
  CAN FD Unpack/1 -> East_Speed/1
  CAN FD Unpack/4 -> Pitch_Angle/1
  CAN FD Unpack/3 -> North_Speed/1
  CAN FD Unpack/6 -> To_Ground_Speed/1
  CAN FD Unpack/5 -> Roll_Angle/1

== system E55_1030/Function-Call Subsystem2/Subsystem19/Enabled Subsystem ==
  In1 : Inport
  In2 : Inport  Port=2
  In3 : Inport  Port=3
  Enable : EnablePort
  CAN FD Unpack : canfdmsglib/CAN FD Unpack  MsgList=(none)  MsgName=INS_0_IMU  ProtocolMode=CAN FD  MsgIDType=Standard (11-bit identifier)  MsgIdentifier=252  MsgLength=64  SignalInfo={ 'INS_IMUAccrnX', '80', '18', 'BE', 'unsigned', 'Standard', '0', '0.0003', '-39', '-39', '39'; 'INS_IMUAccrnY', '144', '18', 'BE', 'unsigned', 'Standard', '0', '0.0003', '-39', '-39', '39'; 'INS_IMUAccrnZ', '208', '18', 'BE', 'unsigned', 'Standard', '0', '0.0003', '-39', '-39', '39'; 'INS_IMUAglRateX', '104', '18', 'BE', 'unsigned', 'Standard', '0', '0.0019074', '-250', '-250', '250.0001'; 'INS_IMUAglRateY', '168', '18', 'BE', 'unsigned', 'Standard', '0', '0.0019074', '-250', '-250', '250.0001'; 'INS_IMUAglRateZ', '232', '18', 'BE', 'unsigned', 'Standard', '0', '0.0019074', '-250', '-250', '250.0001' }  IDPort=off  TimestampPort=off  ErrorPort=off  RemotePort=off  LengthPort=off  StatusPort=off  BRSPort=off  ESIPort=off  DLCPort=off  ApplyMinMax=off
      settings: SourceProductName=Vehicle Network Toolbox  SourceProductBaseCode=VN  DataFormat=manually specified signals
  CANFDUnPackMessage : ec311lib/RapidECU_U34/04CANFDCommunication/CANFDUnPackMessage  mtype=0
      settings: SourceProductName=ECUCoder for S32K311
  INS_IMUAccrnX : Outport
  INS_IMUAccrnY : Outport  Port=2
  INS_IMUAccrnZ : Outport  Port=3
  INS_IMUAglRateX : Outport  Port=4
  INS_IMUAglRateY : Outport  Port=5
  INS_IMUAglRateZ : Outport  Port=6
  wires:
  In1/1 -> CANFDUnPackMessage/1
  In2/1 -> CANFDUnPackMessage/2
  In3/1 -> CANFDUnPackMessage/3
  CANFDUnPackMessage/1 -> CAN FD Unpack/1
  CAN FD Unpack/1 -> INS_IMUAccrnX/1
  CAN FD Unpack/2 -> INS_IMUAccrnY/1
  CAN FD Unpack/3 -> INS_IMUAccrnZ/1
  CAN FD Unpack/5 -> INS_IMUAglRateY/1
  CAN FD Unpack/4 -> INS_IMUAglRateX/1
  CAN FD Unpack/6 -> INS_IMUAglRateZ/1

== system E55_1030/Function-Call Subsystem2/Subsystem2/Enabled Subsystem ==
  In1 : Inport
  In2 : Inport  Port=2
  Enable : EnablePort
  CAN Unpack : canmsglib/CAN Unpack  MsgList=(none)  MsgName=MCU4_287  MsgIDType=Standard (11-bit identifier)  MsgIdentifier=647  MsgLength=8  SignalInfo={ 'MCU4_288_ActualVelocity', '16', '16', 'LE', 'signed', 'Standard', '0', '1', '0', '-32768', '32767'; 'MCU4_288_Error', '9', '1', 'LE', 'unsigned', 'Standard', '0', '1', '0', '0', '1'; 'MCU4_288_ManetizingCurrent', '48', '16', 'LE', 'signed', 'Standard', '0', '0.001', '0', '-20', '20'; 'MCU4_288_TorqueCurrent', '32', '16', 'LE', 'signed', 'Standard', '0', '0.001', '0', '-20', '20' }  IDPort=off  TimestampPort=off  ErrorPort=off  RemotePort=off  LengthPort=off  StatusPort=off  ApplyMinMax=off
      settings: SourceProductName=Vehicle Network Toolbox  SourceProductBaseCode=VN
  CANUnPackMessage : ec311lib/RapidECU_U34/03CANCommunication/CANUnPackMessage  datalength=8  canmessagetype=Standard(11-bit ID)  sampletime=-1
      settings: SourceProductName=ECUCoder for S32K311
  287_ActualVelocity : Outport
  287_Error : Outport  Port=2
  287_Id : Outport  Port=3
  287_Iq : Outport  Port=4
  wires:
  CANUnPackMessage/1 -> CAN Unpack/1
  In2/1 -> CANUnPackMessage/2
  In1/1 -> CANUnPackMessage/1
  CAN Unpack/1 -> 287_ActualVelocity/1
  CAN Unpack/2 -> 287_Error/1
  CAN Unpack/3 -> 287_Id/1
  CAN Unpack/4 -> 287_Iq/1

== system E55_1030/Function-Call Subsystem2/Subsystem3/Enabled Subsystem ==
  In1 : Inport
  In2 : Inport  Port=2
  Enable : EnablePort
  CAN Unpack : canmsglib/CAN Unpack  MsgList=(none)  MsgName=MCU4_283  MsgIDType=Standard (11-bit identifier)  MsgIdentifier=643  MsgLength=8  SignalInfo={ 'MCU4_283_ActualVelocity', '16', '16', 'LE', 'signed', 'Standard', '0', '1', '0', '-32768', '32767'; 'MCU4_283_Error', '9', '1', 'LE', 'unsigned', 'Standard', '0', '1', '0', '0', '1'; 'MCU4_283_ManetizingCurrent', '48', '16', 'LE', 'signed', 'Standard', '0', '0.001', '0', '-20', '20'; 'MCU4_283_TorqueCurrent', '32', '16', 'LE', 'signed', 'Standard', '0', '0.001', '0', '-20', '20' }  IDPort=off  TimestampPort=off  ErrorPort=off  RemotePort=off  LengthPort=off  StatusPort=off  ApplyMinMax=off
      settings: SourceProductName=Vehicle Network Toolbox  SourceProductBaseCode=VN
  CANUnPackMessage : ec311lib/RapidECU_U34/03CANCommunication/CANUnPackMessage  datalength=8  canmessagetype=Standard(11-bit ID)  sampletime=-1
      settings: SourceProductName=ECUCoder for S32K311
  283_ActualVelocity : Outport
  283_Error : Outport  Port=2
  283_Id : Outport  Port=3
  283_Iq : Outport  Port=4
  wires:
  CANUnPackMessage/1 -> CAN Unpack/1
  In2/1 -> CANUnPackMessage/2
  In1/1 -> CANUnPackMessage/1
  CAN Unpack/1 -> 283_ActualVelocity/1
  CAN Unpack/2 -> 283_Error/1
  CAN Unpack/3 -> 283_Id/1
  CAN Unpack/4 -> 283_Iq/1

== system E55_1030/Function-Call Subsystem2/Subsystem4/Enabled Subsystem ==
  In1 : Inport
  In2 : Inport  Port=2
  Enable : EnablePort
  CAN Unpack : canmsglib/CAN Unpack  MsgList=(none)  MsgName=MCU4_288  MsgIDType=Standard (11-bit identifier)  MsgIdentifier=648  MsgLength=8  SignalInfo={ 'MCU4_288_ActualVelocity', '16', '16', 'LE', 'signed', 'Standard', '0', '1', '0', '-32768', '32767'; 'MCU4_288_Error', '9', '1', 'LE', 'unsigned', 'Standard', '0', '1', '0', '0', '1'; 'MCU4_288_ManetizingCurrent', '48', '16', 'LE', 'signed', 'Standard', '0', '0.001', '0', '-20', '20'; 'MCU4_288_TorqueCurrent', '32', '16', 'LE', 'signed', 'Standard', '0', '0.001', '0', '-20', '20' }  IDPort=off  TimestampPort=off  ErrorPort=off  RemotePort=off  LengthPort=off  StatusPort=off  ApplyMinMax=off
      settings: SourceProductName=Vehicle Network Toolbox  SourceProductBaseCode=VN
  CANUnPackMessage : ec311lib/RapidECU_U34/03CANCommunication/CANUnPackMessage  datalength=8  canmessagetype=Standard(11-bit ID)  sampletime=-1
      settings: SourceProductName=ECUCoder for S32K311
  288_ActualVelocity : Outport
  288_Error : Outport  Port=2
  288_Id : Outport  Port=3
  288_Iq : Outport  Port=4
  wires:
  CANUnPackMessage/1 -> CAN Unpack/1
  In2/1 -> CANUnPackMessage/2
  In1/1 -> CANUnPackMessage/1
  CAN Unpack/1 -> 288_ActualVelocity/1
  CAN Unpack/2 -> 288_Error/1
  CAN Unpack/3 -> 288_Id/1
  CAN Unpack/4 -> 288_Iq/1

== system E55_1030/Function-Call Subsystem2/Subsystem5/Enabled Subsystem ==
  In1 : Inport
  In2 : Inport  Port=2
  Enable : EnablePort
  CAN Unpack5 : canmsglib/CAN Unpack  MsgList=(none)  MsgName=MCU4_286  MsgIDType=Standard (11-bit identifier)  MsgIdentifier=646  MsgLength=8  SignalInfo={ 'MCU4_286_ErrorInfo', '32', '16', 'LE', 'unsigned', 'Standard', '0', '1', '0', '0', '65535'; 'MCU4_286_TempIGBT', '48', '16', 'LE', 'signed', 'Standard', '0', '0.1', '0', '-3276.8', '3276.7'; 'MCU4_286_TempInverter', '16', '16', 'LE', 'signed', 'Standard', '0', '0.1', '0', '-3276.8', '3276.7'; 'MCU4_286_TempMotor', '0', '16', 'LE', 'signed', 'Standard', '0', '0.1', '0', '-3276.8', '3276.7' }  IDPort=off  TimestampPort=off  ErrorPort=off  RemotePort=off  LengthPort=off  StatusPort=off  ApplyMinMax=off
      settings: SourceProductName=Vehicle Network Toolbox  SourceProductBaseCode=VN
  CANUnPackMessage5 : ec311lib/RapidECU_U34/03CANCommunication/CANUnPackMessage  datalength=8  canmessagetype=Standard(11-bit ID)  sampletime=-1
      settings: SourceProductName=ECUCoder for S32K311
  ErrorInfo : Outport
  TempIGBT : Outport  Port=2
  TempInverter : Outport  Port=3
  TempMotor : Outport  Port=4
  wires:
  In2/1 -> CANUnPackMessage5/2
  In1/1 -> CANUnPackMessage5/1
  CAN Unpack5/1 -> ErrorInfo/1
  CAN Unpack5/2 -> TempIGBT/1
  CAN Unpack5/4 -> TempMotor/1
  CAN Unpack5/3 -> TempInverter/1
  CANUnPackMessage5/1 -> CAN Unpack5/1

== system E55_1030/Function-Call Subsystem2/Subsystem6/Enabled Subsystem ==
  In1 : Inport
  In2 : Inport  Port=2
  Enable : EnablePort
  CAN Unpack6 : canmsglib/CAN Unpack  MsgList=(none)  MsgName=MCU4_289  MsgIDType=Standard (11-bit identifier)  MsgIdentifier=649  MsgLength=8  SignalInfo={ 'MCU4_289_ErrorInfo', '32', '16', 'LE', 'unsigned', 'Standard', '0', '1', '0', '0', '65535'; 'MCU4_289_TempIGBT', '48', '16', 'LE', 'signed', 'Standard', '0', '0.1', '0', '-3276.8', '3276.7'; 'MCU4_289_TempInverter', '16', '16', 'LE', 'signed', 'Standard', '0', '0.1', '0', '-3276.8', '3276.7'; 'MCU4_289_TempMotor', '0', '16', 'LE', 'signed', 'Standard', '0', '0.1', '0', '-3276.8', '3276.7' }  IDPort=off  TimestampPort=off  ErrorPort=off  RemotePort=off  LengthPort=off  StatusPort=off  ApplyMinMax=off
      settings: SourceProductName=Vehicle Network Toolbox  SourceProductBaseCode=VN
  CANUnPackMessage6 : ec311lib/RapidECU_U34/03CANCommunication/CANUnPackMessage  datalength=8  canmessagetype=Standard(11-bit ID)  sampletime=-1
      settings: SourceProductName=ECUCoder for S32K311
  ErrorInfo : Outport
  TempIGBT : Outport  Port=2
  TempInverter : Outport  Port=3
  TempMotor : Outport  Port=4
  wires:
  In2/1 -> CANUnPackMessage6/2
  In1/1 -> CANUnPackMessage6/1
  CAN Unpack6/1 -> ErrorInfo/1
  CAN Unpack6/2 -> TempIGBT/1
  CAN Unpack6/4 -> TempMotor/1
  CAN Unpack6/3 -> TempInverter/1
  CANUnPackMessage6/1 -> CAN Unpack6/1

== system E55_1030/Function-Call Subsystem2/Subsystem7/Enabled Subsystem ==
  In1 : Inport
  In2 : Inport  Port=2
  Enable : EnablePort
  CAN Unpack7 : canmsglib/CAN Unpack  MsgList=(none)  MsgName=MCU4_28A  MsgIDType=Standard (11-bit identifier)  MsgIdentifier=650  MsgLength=8  SignalInfo={ 'MCU4_28A_ErrorInfo', '32', '16', 'LE', 'unsigned', 'Standard', '0', '1', '0', '0', '65535'; 'MCU4_28A_TempIGBT', '48', '16', 'LE', 'signed', 'Standard', '0', '0.1', '0', '-3276.8', '3276.7'; 'MCU4_28A_TempInverter', '16', '16', 'LE', 'signed', 'Standard', '0', '0.1', '0', '-3276.8', '3276.7'; 'MCU4_28A_TempMotor', '0', '16', 'LE', 'signed', 'Standard', '0', '0.1', '0', '-3276.8', '3276.7' }  IDPort=off  TimestampPort=off  ErrorPort=off  RemotePort=off  LengthPort=off  StatusPort=off  ApplyMinMax=off
      settings: SourceProductName=Vehicle Network Toolbox  SourceProductBaseCode=VN
  CANUnPackMessage7 : ec311lib/RapidECU_U34/03CANCommunication/CANUnPackMessage  datalength=8  canmessagetype=Standard(11-bit ID)  sampletime=-1
      settings: SourceProductName=ECUCoder for S32K311
  ErrorInfo : Outport
  TempIGBT : Outport  Port=2
  TempInverter : Outport  Port=3
  TempMotor : Outport  Port=4
  wires:
  In2/1 -> CANUnPackMessage7/2
  In1/1 -> CANUnPackMessage7/1
  CAN Unpack7/1 -> ErrorInfo/1
  CAN Unpack7/2 -> TempIGBT/1
  CAN Unpack7/4 -> TempMotor/1
  CAN Unpack7/3 -> TempInverter/1
  CANUnPackMessage7/1 -> CAN Unpack7/1

== system E55_1030/Function-Call Subsystem2/Subsystem8/Enabled Subsystem ==
  In1 : Inport
  In2 : Inport  Port=2
  Enable : EnablePort
  CAN Unpack9 : canmsglib/CAN Unpack  MsgList=(none)  MsgName=IVT_Msg_Result_W  MsgIDType=Standard (11-bit identifier)  MsgIdentifier=1318  MsgLength=6  SignalInfo={ 'IVT_MsgCount', '8', '4', 'LE', 'unsigned', 'Standard', '0', '1', '0', '0', '15'; 'IVT_Msg_Result_W', '40', '32', 'BE', 'signed', 'Standard', '0', '1', '0', '-12000', '80000' }  IDPort=off  TimestampPort=off  ErrorPort=off  RemotePort=off  LengthPort=off  StatusPort=off  ApplyMinMax=off
      settings: SourceProductName=Vehicle Network Toolbox  SourceProductBaseCode=VN
  CANUnPackMessage8 : ec311lib/RapidECU_U34/03CANCommunication/CANUnPackMessage  datalength=6  canmessagetype=Standard(11-bit ID)  sampletime=-1
      settings: SourceProductName=ECUCoder for S32K311
  IVT_MsgCount : Outport
  IVT_Msg_Result_W : Outport  Port=2
  wires:
  In2/1 -> CANUnPackMessage8/2
  In1/1 -> CANUnPackMessage8/1
  CANUnPackMessage8/1 -> CAN Unpack9/1
  CAN Unpack9/1 -> IVT_MsgCount/1
  CAN Unpack9/2 -> IVT_Msg_Result_W/1
